simulink model "DeVriesSlipModelRW"  (R2017b)
settings: Solver=VariableStepAuto  StartTime=0.0  StopTime=100  RelTol=1e-3
undefined symbols (not defined in the file): b_contact, C_F_alpha, C_F_kappa, Cylinder, epsilon, g, k_contact, lengthRW, mR, Parts_Lib, radiusRW, rhoRW, sigma, X, xPla, Y, yPla, Z
libraries: nesl_utility x16, sm_lib x11, Contact_Forces_Lib x8, vrlib x2, dspsrcs4 x1, simulink x1
settings Model: Creator=r_ahmed_afzal  LastModifiedBy=r_ahmed_afzal
settings SolverCC: ZeroCrossAlgorithm=Adaptive

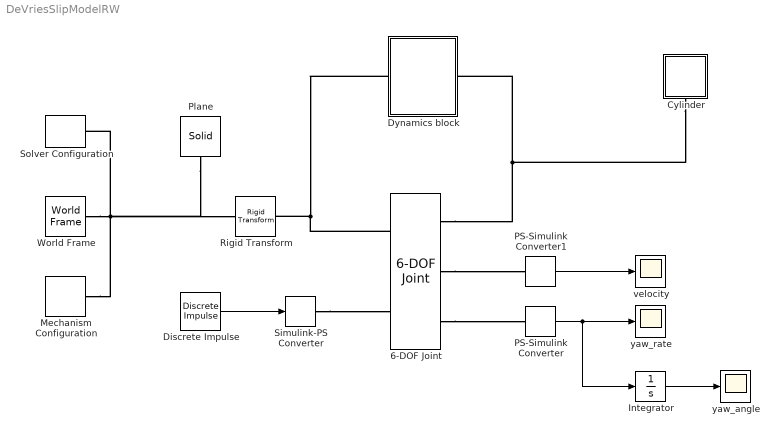
== system DeVriesSlipModelRW ==
  6-DOF Joint : sm_lib/Joints/6-DOF Joint  SenseConstraintForce=off  SenseConstraintForceX=off  SenseConstraintForceY=off  SenseConstraintForceZ=off  SenseConstraintTorque=off  SenseConstraintTorqueX=off  SenseConstraintTorqueY=off  SenseConstraintTorqueZ=off  SenseTotalForce=off  SenseTotalForceX=off  SenseTotalForceY=off  SenseTotalForceZ=off  SenseTotalTorque=off  SenseTotalTorqueX=off  SenseTotalTorqueY=off  SenseTotalTorqueZ=off  CompositeWrenchDir=FollowerOnBase  CompositeWrenchFrame=BaseFrame  PxEquilibriumPosition=0  PxEquilibriumPositionUnits=m  PxSpringStiffness=0  PxSpringStiffnessUnits=N/m  PxDampingCoefficient=0  PxDampingCoefficientUnits=N/(m/s)  PxTorqueActuationMode=NoTorque  PxMotionActuationMode=ComputedMotion  PxSensePosition=off  PxSenseVelocity=off  PxSenseAcceleration=off  PxSenseTorqueForce=off  PxPositionTargetSpecify=on  PxPositionTargetPriority=High  PxPositionTargetValue=radiusRW  PxPositionTargetValueUnits=m  PxVelocityTargetSpecify=off  PxVelocityTargetPriority=High  PxVelocityTargetValue=0  PxVelocityTargetValueUnits=m/s  PyEquilibriumPosition=0  PyEquilibriumPositionUnits=m  PySpringStiffness=0  PySpringStiffnessUnits=N/m  PyDampingCoefficient=0  PyDampingCoefficientUnits=N/(m/s)  PyTorqueActuationMode=NoTorque  PyMotionActuationMode=ComputedMotion  PySensePosition=off  PySenseVelocity=on  PySenseAcceleration=off  PySenseTorqueForce=off  PyPositionTargetSpecify=on  PyPositionTargetPriority=High  PyPositionTargetValue=-xPla/2 + 0.1  PyPositionTargetValueUnits=m  PyVelocityTargetSpecify=on  PyVelocityTargetPriority=High  PyVelocityTargetValue=v0  PyVelocityTargetValueUnits=m/s  PzEquilibriumPosition=0  PzEquilibriumPositionUnits=m  PzSpringStiffness=0  PzSpringStiffnessUnits=N/m  PzDampingCoefficient=0  PzDampingCoefficientUnits=N/(m/s)  PzTorqueActuationMode=NoTorque  PzMotionActuationMode=ComputedMotion  PzSensePosition=off  PzSenseVelocity=off  PzSenseAcceleration=off  PzSenseTorqueForce=off  PzPositionTargetSpecify=off  PzPositionTargetPriority=High  PzPositionTargetValue=0  PzPositionTargetValueUnits=m  PzVelocityTargetSpecify=off  PzVelocityTargetPriority=High  PzVelocityTargetValue=0  PzVelocityTargetValueUnits=m/s  SphDefPosRotationMethod=None  SphDefPosRotationAngleUnits=deg  SphDefPosRotationStandardAxis=+Z  SphDefPosRotationAngle=0.0  SphDefPosRotationArbitraryAxis=[0 0 1]  SphDefPosFollAlignAxisA=+X  SphDefPosBaseAlignAxisA=+Y  SphDefPosFollAlignAxisB=+Y  SphDefPosBaseAlignAxisB=+Z  SphDefPosRotationSequenceAxes=FollowerAxes  SphDefPosRotationSequence=XYX  SphDefPosRotationSequenceAngles=[0 0 0]  SphDefPosRotationSequenceAnglesUnits=deg  SphDefPosRotationMatrix=[1 0 0; 0 1 0; 0 0 1]  SphEqPosRotationMethod=None  SphEqPosRotationAngleUnits=deg  SphEqPosRotationStandardAxis=+Z  SphEqPosRotationAngle=0.0  SphEqPosRotationArbitraryAxis=[0 0 1]  SphEqPosFollAlignAxisA=+X  SphEqPosBaseAlignAxisA=+Y  SphEqPosFollAlignAxisB=+Y  SphEqPosBaseAlignAxisB=+Z  SphEqPosRotationSequenceAxes=FollowerAxes  SphEqPosRotationSequence=XYX  SphEqPosRotationSequenceAngles=[0 0 0]  SphEqPosRotationSequenceAnglesUnits=deg  SphEqPosRotationMatrix=[1 0 0; 0 1 0; 0 0 1]  SphSpringStiffness=0  SphSpringStiffnessUnits=N*m/deg  SphDampingCoefficient=0  SphDampingCoefficientUnits=N*m/(deg/s)  SphActuateTorqueX=off  SphActuateTorqueY=off  SphActuateTorqueZ=on  SphActuateTorque=off  SphTorqueActuationMode=InputTorque  SphMotionActuationMode=ComputedMotion  SphActuationFrame=FollowerFrame  SphSensePosition=off  SphSenseVelocityX=on  SphSenseVelocityY=off  SphSenseVelocityZ=off  SphSenseVelocity=off  SphSenseAccelerationX=off  SphSenseAccelerationY=off  SphSenseAccelerationZ=off  SphSenseAcceleration=off  SphSenseTorqueX=off  SphSenseTorqueY=off  SphSenseTorqueZ=off  SphSenseTorqueForce=off  SphSensingFrame=BaseFrame  SphPositionTargetRotationMethod=None  SphPositionTargetRotationAngleUnits=deg  SphPositionTargetRotationStandardAxis=+Z  SphPositionTargetRotationAngle=0.0  SphPositionTargetRotationArbitraryAxis=[0 0 1]  SphPositionTargetFollAlignAxisA=+X  SphPositionTargetBaseAlignAxisA=+Y  SphPositionTargetFollAlignAxisB=+Y  SphPositionTargetBaseAlignAxisB=+Z  SphPositionTargetRotationSequenceAxes=FollowerAxes  SphPositionTargetRotationSequence=XYX  SphPositionTargetRotationSequenceAngles=[0 0 0]  SphPositionTargetRotationSequenceAnglesUnits=deg  SphPositionTargetRotationMatrix=[1 0 0; 0 1 0; 0 0 1]  SphPositionTargetSpecify=off  SphPositionTargetPriority=High  SphVelocityTargetValue=[0 0 0]  SphVelocityTargetValueUnits=deg/s  SphVelocityTargetSpecify=off  SphVelocityTargetPriority=High  SphVelocityTargetInFollowerFrame=on
  Cylinder : Subsystem  Tag=CustomStyle  AncestorBlock=Parts_Lib/Cylinder  mask(Solid Cylinder with Markings){cyl_radius=radiusRW, cyl_length=lengthRW, cyl_density=rhoRW, cyl_color=blue, cyl_opacity=1, cyl_color_custom=[0.7920    0.9900    0.9900], mark_radius=[0.75 0.5], mark_len_factor=1.01, mark_angle=60, mark_color=purple, mark_opacity=1}
      mask prompts: cyl_radius "Radius (m)"; cyl_length "Length (m)"; cyl_density "Density (kg/m^3)"; cyl_color "Color"; cyl_opacity "Opacity (0-1)"; cyl_color_custom "Custom Color (rgb)"; mark_radius "Outer, inner radius (% of cylinder radius)"; mark_len_factor "Length (factor of cylinder length)"; mark_angle "Sweep angle (deg)"; mark_color "Color"; mark_opacity "Opacity (0-1)"
      mask init:
      | curblk = gcb;
      | if strcmp(get_param(curblk,'cyl_color'),'red')
      |     set_param([curblk '/Cylinder'],'GraphicDiffuseColor','[0.8 0.0 0.2]');
      |     set_param(curblk,'BackGroundColor','[0.901961, 0.396078, 0.396078]');
      | elseif strcmp(get_param(gcb,'cyl_color'),'blue')
      |     set_param([curblk '/Cylinder'],'GraphicDiffuseColor','[0.0 0.5 0.7]');
      |     set_param(curblk,'BackGroundColor','[0.541176, 0.698039, 0.901961]');
      | elseif strcmp(get_param(gcb,'cyl_color'),'yellow')
      |     set_param([curblk '/Cylinder'],'GraphicDiffuseColor','[1.0 1.0 0.0]');
      |     set_param(curblk,'BackGroundColor','[0.905882, 0.890196, 0.392157]');
      | elseif strcmp(get_param(gcb,'cyl_color'),'gray')
      |     set_param([curblk '/Cylinder'],'GraphicDiffuseColor','[1.0 1.0 1.0]*0.6');
      |     set_param(curblk,'BackGroundColor','[0.6 0.6 0.6]');
      | elseif strcmp(get_param(gcb,'cyl_color'),'custom')
      |     set_param([curblk '/Cylinder'],'GraphicDiffuseColor',get_param(curblk,'cyl_color_custom'));
      |     set_param(curblk,'BackGroundColor','[1 1 1]');
      | end
      | 
      | if strcmp(get_param(curblk,'mark_color'),'purple')
      |     set_param([curblk '/Vis1'],'GraphicDiffuseColor','[0.4 0.0 0.4]');
      |     set_param([curblk '/Vis2'],'GraphicDiffuseColor','[0.4 0.0 0.4]');
      | elseif strcmp(get_param(gcb,'mark_color'),'green')
      |     set_param([curblk '/Vis1'],'GraphicDiffuseColor','[0.0 0.8 0.0]');
      |     set_param([curblk '/Vis2'],'GraphicDiffuseColor','[0.0 0.8 0.0]');
      | elseif strcmp(get_param(gcb,'mark_color'),'orange')
      |     set_param([curblk '/Vis1'],'GraphicDiffuseColor','[1.0 0.6 0.0]');
      |     set_param([curblk '/Vis2'],'GraphicDiffuseColor','[1.0 0.6 0.0]');
      | elseif strcmp(get_param(gcb,'mark_color'),'black')
      |     set_param([curblk '/Vis1'],'GraphicDiffuseColor','[0.0 0.0 0.0]');
      |     set_param([curblk '/Vis2'],'GraphicDiffuseColor','[0.0 0.0 0.0]');
      | end
      | 
      | clear curblk
      mask TypeOptions cyl_color: red | gray | yellow | blue | custom
      mask Callback cyl_color:
      | maskObj = Simulink.Mask.get(gcb);
      | clr_h = maskObj.getParameter('cyl_color_custom');
      | if strcmp(get_param(gcb,'cyl_color'),'custom')
      |     clr_h.Visible = 'on';
      | else
      |     clr_h.Visible = 'off';
      | end
      mask TypeOptions mark_color: purple | green | orange | black
      mask DialogControl Container4 Prompt: Cylinder
      mask DialogControl Container7 Prompt: Markings
  Discrete Impulse : dspsrcs4/Discrete  Impulse  Delay=100  SampleTime=1  FrameSample=1  OutputFrames=off  dataType=double  isSigned=on  wordLen=16  udDataType=sfix(16)  fracBitsMode=Best precision  numFracBits=15  OutDataTypeStr=double  LastOutDataTypeStr=double
  Dynamics block : Subsystem
  Integrator : Integrator
  Mechanism Configuration : sm_lib/Utilities/Mechanism Configuration  UniformGravity=Constant  GravityVector=[0 0 -g]  GravityUnits=m/s^2  LinearizationDelta=0.001
  PS-Simulink Converter : nesl_utility/PS-Simulink Converter  PhysicalDomain=network_engine_domain  SubClassName=ps_output  LeftPortType=input  RightPortType=output  PseudoPeriodic=off  Frequencies=[]  Unit=1  AffineConversion=off
  PS-Simulink Converter1 : nesl_utility/PS-Simulink Converter  PhysicalDomain=network_engine_domain  SubClassName=ps_output  LeftPortType=input  RightPortType=output  PseudoPeriodic=off  Frequencies=[]  Unit=1  AffineConversion=off
  Plane : sm_lib/Body Elements/Solid  InertiaType=CalculateFromGeometry  Mass=1  MassUnits=kg  CenterOfMass=[0 0 0]  CenterOfMassUnits=m  MomentsOfInertia=[1 1 1]  MomentsOfInertiaUnits=kg*m^2  ProductsOfInertia=[1 1 1]  ProductsOfInertiaUnits=kg*m^2  DensityBased=on  Density=1000  DensityUnits=kg/m^3  DoExposeReferenceFrame=on  SerializedFrames=<Frames/>  GraphicType=FromGeometry  MarkerShape=Sphere  MarkerSize=10  GraphicVisPropType=SimpleVisualProperties  GraphicDiffuseColor=[0.5 0.5 0.5]  GraphicSpecularColor=[0.5 0.5 0.5 1.0]  GraphicAmbientColor=[0.15 0.15 0.15 1.0]  GraphicEmissiveColor=[0.0 0.0 0.0 1.0]  GraphicShininess=75  GraphicOpacity=0.5  GeometryShape=Brick  RectangleSize=[1 1]  RectangleSizeUnits=m  BrickDimensions=[xPla yPla 0.01]  BrickDimensionUnits=m  CylinderRadius=1  CylinderRadiusUnits=m  CylinderLength=1  CylinderLengthUnits=m  SphereRadius=1  SphereRadiusUnits=m  EllipsoidRadii=[1 1 1]  EllipsoidRadiiUnits=m  ExtrusionCrossSection=[1 1; -1 1; -1 -1; 1 -1]  ExtrusionCrossSectionUnits=m  ExtrusionLength=1  ExtrusionLengthUnits=m  PolygonNumSides=3  PolygonOuterRadius=1  PolygonOuterRadiusUnits=m  ExtGeomFileType=STEP  ExtGeomFileUnits=m  RevolutionCrossSection=[1 1; 1 -1; 2 -1; 2 1]  RevolutionCrossSectionUnits=m  RevolutionExtent=Full  RevolutionAngle=180  RevolutionAngleUnits=deg
  Rigid Transform : sm_lib/Frames and Transforms/Rigid Transform  TranslationMethod=None  TranslationStandardOffset=0  TranslationLengthUnit=m  TranslationStandardAxis=+Z  TranslationCartesianOffset=[0 0 0]  TranslationROffset=0  TranslationROffsetUnits=m  TranslationZOffset=0  TranslationZOffsetUnits=m  TranslationThetaOffset=0  TranslationThetaOffsetUnits=deg  RotationMethod=AlignedAxes  RotationAngleUnits=deg  RotationStandardAxis=+Z  RotationAngle=0.0  RotationArbitraryAxis=[0 0 1]  FollAlignAxisA=+Z  BaseAlignAxisA=+Y  FollAlignAxisB=+Y  BaseAlignAxisB=+X  RotationSequenceAxes=FollowerAxes  RotationSequence=XYX  RotationSequenceAngles=[0 0 0]  RotationSequenceAnglesUnits=deg  RotationMatrix=[1 0 0; 0 1 0; 0 0 1]
  Simulink-PS Converter : nesl_utility/Simulink-PS Converter  PhysicalDomain=network_engine_domain  SubClassName=ps_input  LeftPortType=input  RightPortType=output  PseudoPeriodic=off  Frequencies=[]  NoiseDistribution=none  NoiseParameters=[]  Unit=1  AffineConversion=off  FilteringAndDerivatives=provide  SimscapeFilterOrder=1  InputFilterTimeConstant=0.001  UdotUserProvided=0
  Solver Configuration : nesl_utility/Solver Configuration  PhysicalDomain=network_engine_domain  SubClassName=solver  LeftPortType=input  RightPortType=generic  Accelerate=off  Tones=[]  Harmonics=[]  SimulateNoise=off  Profile=off  UseLocalSampling=off  EnableSwitchedLinearOptims=on  FrequencyDomain=off  UseCCode=off  RelTol=0.001  AbsTol=1e-06  MinStep=1e-09  ToWorkspace=off  RevertToSquareIcSolve=off  NumHomotopyIterations=100  PhasorMode=off  PhasorModeNumHarmonics=1  DoDC=off  ResidualTolerance=1e-09  UseLocalSolver=off  LocalSolverChoice=NE_BACKWARD_EULER_ADVANCER  LocalSolverSampleTime=0.001  DoFixedCost=off  MaxNonlinIter=3  MaxModeIter=2  LinearAlgebra=Sparse  DelaysMemoryBudget=1024  AutomaticFiltering=on  FilteringTimeConstant=0.001
  World Frame : sm_lib/Frames and Transforms/World Frame
  velocity : Scope
  yaw_angle : Scope
  yaw_rate : Scope
  wires:
  Integrator/1 -> yaw_angle/1
  PS-Simulink Converter1/1 -> velocity/1
  PS-Simulink Converter/1 -> Integrator/1, yaw_rate/1
  Discrete Impulse/1 -> Simulink-PS Converter/1
  connections:
  Mechanism Configuration/RConn1 -- World Frame/RConn1 -- Rigid Transform/LConn1 -- Plane/RConn1 -- Solver Configuration/RConn1
  Dynamics block/LConn1 -- 6-DOF Joint/LConn1 -- Rigid Transform/RConn1
  Cylinder/LConn1 -- 6-DOF Joint/RConn1 -- Dynamics block/RConn1
  6-DOF Joint/RConn2 -- PS-Simulink Converter1/LConn1
  6-DOF Joint/RConn3 -- PS-Simulink Converter/LConn1
  Simulink-PS Converter/RConn1 -- 6-DOF Joint/LConn2

== system DeVriesSlipModelRW/Cylinder ==
  Cylinder : sm_lib/Body Elements/Solid  InertiaType=CalculateFromGeometry  Mass=mR  MassUnits=kg  CenterOfMass=[0 0 0]  CenterOfMassUnits=m  MomentsOfInertia=momentInertiaRW  MomentsOfInertiaUnits=kg*m^2  ProductsOfInertia=[0 0 0]  ProductsOfInertiaUnits=kg*m^2  DensityBased=on  Density=cyl_density  DensityUnits=kg/(m^3)  DoExposeReferenceFrame=on  SerializedFrames=<Frames/>  GraphicType=FromGeometry  MarkerShape=Sphere  MarkerSize=10  MarkerSizeUnits=m  GraphicVisPropType=SimpleVisualProperties  GraphicDiffuseColor=[0.0 0.5 0.7]  GraphicSpecularColor=[0.5 0.5 0.5 1.0]  GraphicAmbientColor=[0.15 0.15 0.15 1.0]  GraphicEmissiveColor=[0.0 0.0 0.0 1.0]  GraphicShininess=75  GraphicOpacity=cyl_opacity  GeometryShape=Cylinder  RectangleSize=[1 1]  RectangleSizeUnits=m  BrickDimensions=[1 1 1]  BrickDimensionUnits=m  CylinderRadius=cyl_radius  CylinderRadiusUnits=m  CylinderLength=cyl_length  CylinderLengthUnits=m  SphereRadius=1  SphereRadiusUnits=m  EllipsoidRadii=[1 1 1]  EllipsoidRadiiUnits=m  ExtrusionCrossSection=[1 1; -1 1; -1 -1; 1 -1]  ExtrusionCrossSectionUnits=m  ExtrusionLength=1  ExtrusionLengthUnits=m  PolygonNumSides=3  PolygonOuterRadius=1  PolygonOuterRadiusUnits=m  ExtGeomFileType=STL  ExtGeomFileUnits=m  RevolutionCrossSection=[1 1; 1 -1; 2 -1; 2 1]  RevolutionCrossSectionUnits=m  RevolutionExtent=Full  RevolutionAngle=180  RevolutionAngleUnits=deg
  Transform Vis2 : sm_lib/Frames and Transforms/Rigid Transform  TranslationMethod=None  TranslationStandardOffset=0  TranslationLengthUnit=m  TranslationStandardAxis=+Z  TranslationCartesianOffset=[0 0 0]  TranslationROffset=0  TranslationROffsetUnits=m  TranslationZOffset=0  TranslationZOffsetUnits=m  TranslationThetaOffset=0  TranslationThetaOffsetUnits=deg  RotationMethod=StandardAxis  RotationAngleUnits=deg  RotationStandardAxis=+Y  RotationAngle=180  RotationArbitraryAxis=[0 0 1]  FollAlignAxisA=+X  BaseAlignAxisA=+Y  FollAlignAxisB=+Y  BaseAlignAxisB=+Z  RotationSequenceAxes=FollowerAxes  RotationSequence=XYX  RotationSequenceAngles=[0 0 0]  RotationSequenceAnglesUnits=deg  RotationMatrix=[1 0 0; 0 1 0; 0 0 1]
  Vis1 : sm_lib/Body Elements/Solid  InertiaType=CalculateFromGeometry  Mass=1  MassUnits=kg  CenterOfMass=[0 0 0]  CenterOfMassUnits=m  MomentsOfInertia=[1 1 1]  MomentsOfInertiaUnits=kg*m^2  ProductsOfInertia=[0 0 0]  ProductsOfInertiaUnits=kg*m^2  DensityBased=on  Density=1e-3  DensityUnits=kg/(m^3)  DoExposeReferenceFrame=on  SerializedFrames=<Frames/>  GraphicType=FromGeometry  MarkerShape=Sphere  MarkerSize=10  MarkerSizeUnits=m  GraphicVisPropType=SimpleVisualProperties  GraphicDiffuseColor=[0.4 0.0 0.4]  GraphicSpecularColor=[0.5 0.5 0.5 1.0]  GraphicAmbientColor=[0.15 0.15 0.15 1.0]  GraphicEmissiveColor=[0.0 0.0 0.0 1.0]  GraphicShininess=75  GraphicOpacity=mark_opacity  GeometryShape=GeneralSolidOfRevolution  RectangleSize=[1 1]  RectangleSizeUnits=m  BrickDimensions=[1 1 1]  BrickDimensionUnits=m  CylinderRadius=0.1  CylinderRadiusUnits=m  CylinderLength=0.01  CylinderLengthUnits=m  SphereRadius=1  SphereRadiusUnits=m  EllipsoidRadii=[1 1 1]  EllipsoidRadiiUnits=m  ExtrusionCrossSection=[1 1; -1 1; -1 -1; 1 -1]  ExtrusionCrossSectionUnits=m  ExtrusionLength=1  ExtrusionLengthUnits=m  PolygonNumSides=3  PolygonOuterRadius=1  PolygonOuterRadiusUnits=m  ExtGeomFileType=STL  ExtGeomFileUnits=m  RevolutionCrossSection=[cyl_radius*mark_radius(1) cyl_length/2*mark_len_factor; cyl_radius*mark_radius(2) cyl_length/2*mark_len_factor; cyl_radius*mark_radius(2) -cyl_length/2*mark_len_factor; cyl_radius*mark_radius(1) -cyl_length/2*mark_len_factor]  RevolutionCrossSectionUnits=m  RevolutionExtent=Custom  RevolutionAngle=mark_angle  RevolutionAngleUnits=deg
  Vis2 : sm_lib/Body Elements/Solid  InertiaType=CalculateFromGeometry  Mass=1  MassUnits=kg  CenterOfMass=[0 0 0]  CenterOfMassUnits=m  MomentsOfInertia=[1 1 1]  MomentsOfInertiaUnits=kg*m^2  ProductsOfInertia=[0 0 0]  ProductsOfInertiaUnits=kg*m^2  DensityBased=on  Density=1e-3  DensityUnits=kg/(m^3)  DoExposeReferenceFrame=on  SerializedFrames=<Frames/>  GraphicType=FromGeometry  MarkerShape=Sphere  MarkerSize=10  MarkerSizeUnits=m  GraphicVisPropType=SimpleVisualProperties  GraphicDiffuseColor=[0.4 0.0 0.4]  GraphicSpecularColor=[0.5 0.5 0.5 1.0]  GraphicAmbientColor=[0.15 0.15 0.15 1.0]  GraphicEmissiveColor=[0.0 0.0 0.0 1.0]  GraphicShininess=75  GraphicOpacity=mark_opacity  GeometryShape=GeneralSolidOfRevolution  RectangleSize=[1 1]  RectangleSizeUnits=m  BrickDimensions=[1 1 1]  BrickDimensionUnits=m  CylinderRadius=0.1  CylinderRadiusUnits=m  CylinderLength=0.01  CylinderLengthUnits=m  SphereRadius=1  SphereRadiusUnits=m  EllipsoidRadii=[1 1 1]  EllipsoidRadiiUnits=m  ExtrusionCrossSection=[1 1; -1 1; -1 -1; 1 -1]  ExtrusionCrossSectionUnits=m  ExtrusionLength=1  ExtrusionLengthUnits=m  PolygonNumSides=3  PolygonOuterRadius=1  PolygonOuterRadiusUnits=m  ExtGeomFileType=STL  ExtGeomFileUnits=m  RevolutionCrossSection=[cyl_radius*mark_radius(1) cyl_length/2*mark_len_factor; cyl_radius*mark_radius(2) cyl_length/2*mark_len_factor; cyl_radius*mark_radius(2) -cyl_length/2*mark_len_factor; cyl_radius*mark_radius(1) -cyl_length/2*mark_len_factor]  RevolutionCrossSectionUnits=m  RevolutionExtent=Custom  RevolutionAngle=mark_angle  RevolutionAngleUnits=deg
  R : PMIOPort  Port=1  Side=Left
  connections:
  R/RConn1 -- Cylinder/RConn1 -- Transform Vis2/LConn1 -- Vis1/RConn1
  Vis2/RConn1 -- Transform Vis2/RConn1

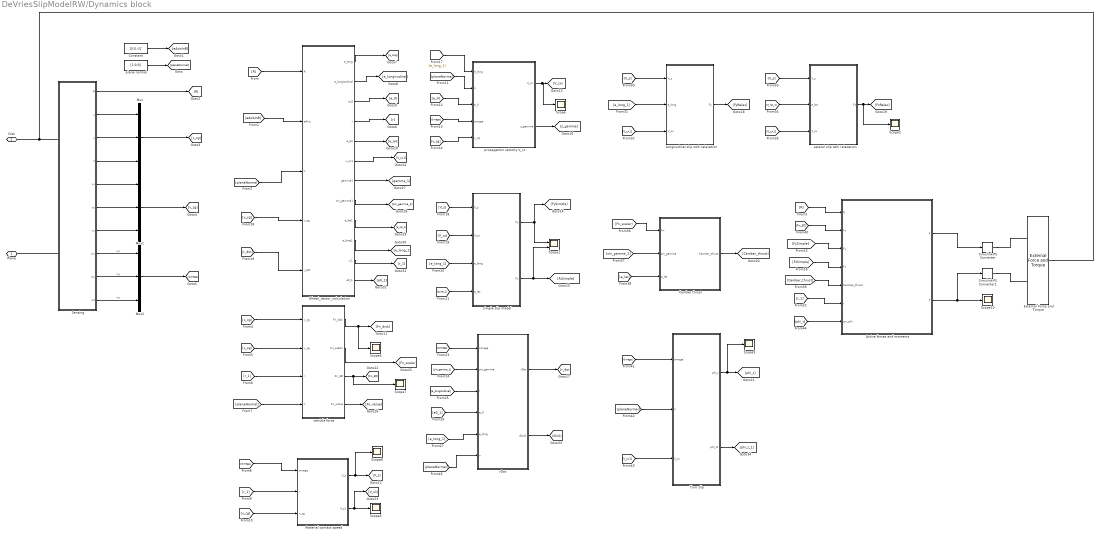
== system DeVriesSlipModelRW/Dynamics block ==
  Active forces and moments : Subsystem
  Camber thrust : Subsystem
  Constant : Constant  Value=[0,0,-1]'
  External Force and Torque : sm_lib/Forces and Torques/External Force and Torque  ForceResolutionFrame=AttachedFrame  EnableForceX=off  EnableForceY=off  EnableForceZ=off  EnableForce=on  TorqueResolutionFrame=AttachedFrame  EnableTorqueX=off  EnableTorqueY=off  EnableTorqueZ=off  EnableTorque=on
  Lateral slip wtih relaxation : Subsystem
  Longitudinal slip wtih relaxation : Subsystem
  Material contact speed : Subsystem
  Mux : Mux  Inputs=3
  Mux1 : Mux  Inputs=3
  Mux2 : Mux  Inputs=3
  Scope{,2,4..7,9..10} (8 alike) : Scope
  Scope1 : Scope  NumInputPorts=2
  Sensing : Subsystem
  Simulink-PS Converter : nesl_utility/Simulink-PS Converter  PhysicalDomain=network_engine_domain  SubClassName=ps_input  LeftPortType=input  RightPortType=output  PseudoPeriodic=off  Frequencies=[]  NoiseDistribution=none  NoiseParameters=[]  Unit=1  AffineConversion=off  FilteringAndDerivatives=provide  SimscapeFilterOrder=1  InputFilterTimeConstant=0.001  UdotUserProvided=0
  Simulink-PS Converter1 : nesl_utility/Simulink-PS Converter  PhysicalDomain=network_engine_domain  SubClassName=ps_input  LeftPortType=input  RightPortType=output  PseudoPeriodic=off  Frequencies=[]  NoiseDistribution=none  NoiseParameters=[]  Unit=1  AffineConversion=off  FilteringAndDerivatives=provide  SimscapeFilterOrder=1  InputFilterTimeConstant=0.001  UdotUserProvided=0
  Turn slip : Subsystem
  Wheel_vector_calculation : Subsystem
  plane normal : Constant  Value=[1;0;0]
  propagation velocity V_cx : Subsystem
  rDot : Subsystem
  simple slip model : Subsystem
  verticle force : Subsystem
  Plane : PMIOPort  Port=1  Side=Left
  Disk : PMIOPort  Port=2  Side=Right
  wires:
  plane normal/1 -> [planeNormal]
  Constant/1 -> [eAxisInB]
  Sensing/1(R) -> [R]
  Sensing/2(x) -> Mux/1
  Sensing/3(y) -> Mux/2
  Sensing/4(z) -> Mux/3
  Mux/1 -> [x_cg]
  Sensing/6(vy) -> Mux1/2
  Sensing/5(vx) -> Mux1/1
  Sensing/7(vz) -> Mux1/3
  Mux1/1 -> [v_cg]
  Sensing/9(wy) -> Mux2/2  "wy"
  Sensing/8(wx) -> Mux2/1  "wx"
  Sensing/10(wz) -> Mux2/3  "wz"
  [R] -> Wheel_vector_calculation/1(R)
  [planeNormal] -> Wheel_vector_calculation/3(n)
  [x_cg] -> verticle force/1(x_cg)
  [v_cg] -> verticle force/2(v_cg)
  Wheel_vector_calculation/4(r) -> [r]
  Wheel_vector_calculation/1(e_long) -> [e_long]
  Wheel_vector_calculation/2(e_longitudinal) -> [e_longitudinal]
  Wheel_vector_calculation/3(e_0) -> [e_0]
  Wheel_vector_calculation/5(e_lat) -> [e_lat]
  [r_1] -> verticle force/3(r)
  [planeNormal] -> verticle force/4(n)
  verticle force/1(Fn_disk) -> Scope4/1, [Fn_disk]
  [Omega] -> Material contact speed/1(omega)
  [r_1] -> Material contact speed/2(r)
  [v_cg] -> Material contact speed/3(v_cg)
  Material contact speed/1(V_s) -> Scope6/1, [V_s]
  [planeNormal] -> propagation velocity V_cx/2(n)
  [e_0] -> propagation velocity V_cx/3(e_0)
  [Omega] -> propagation velocity V_cx/4(omega)
  [v_cg] -> propagation velocity V_cx/5(v_cg)
  [e_long_1] -> propagation velocity V_cx/1(e_long)
  propagation velocity V_cx/1(V_cx) -> Scope/1, [V_cx]
  [V_s] -> simple slip model/1(V_s)
  [V_cx] -> simple slip model/2(V_cx)
  [e_long_1] -> simple slip model/3(e_long)
  [e_lat_1] -> simple slip model/4(e_lat)
  simple slip model/2(Fz) -> Scope1/2, [FzSimple]
  [Omega] -> rDot/1(omega)
  propagation velocity V_cx/2(s_gamma) -> [s_gamma]
  [sin_gamma_1] -> rDot/2(sin_gamma)
  [e_longitudinal] -> rDot/3(l)
  [e0_1] -> rDot/4(e_0)
  [e_long_1] -> rDot/5(e_long)
  simple slip model/1(Fy) -> [FySimple], Scope1/1
  [V_s] -> Longitudinal slip wtih relaxation/1(V_s)
  [e_long_1] -> Longitudinal slip wtih relaxation/2(e_long)
  [V_cx1] -> Longitudinal slip wtih relaxation/3(V_cx)
  [e_lat_1] -> Lateral slip wtih relaxation/2(e_lat)
  [V_s] -> Lateral slip wtih relaxation/1(V_s)
  [V_cx1] -> Lateral slip wtih relaxation/3(V_cx)
  Longitudinal slip wtih relaxation/1(Fy) -> [FyRelax]
  Lateral slip wtih relaxation/1(Fz) -> Scope2/1, [FzRelax]
  [Fn_scalar] -> Camber thrust/1(Fn)
  [sin_gamma_1] -> Camber thrust/2(sin_gamma)
  [e_lat] -> Camber thrust/3(e_lat)
  Camber thrust/1(Camber_thrust) -> [Camber_thrust]
  Turn slip/1(phi_t) -> Scope9/1, [phi_t]
  [V_cx1] -> Turn slip/3(V_cx)
  [planeNormal] -> Turn slip/2(n)
  [Omega] -> Turn slip/1(omega)
  [R] -> Active forces and moments/1(R)
  [Fn_3D] -> Active forces and moments/2(Fx)
  [FySimple] -> Active forces and moments/3(Fy)
  [r_1] -> Active forces and moments/6(r)
  Active forces and moments/1(F) -> Simulink-PS Converter/1
  Active forces and moments/2(T) -> Scope10/1, Simulink-PS Converter1/1
  verticle force/3(Fn_3D) -> [Fn_3D], Scope7/1
  verticle force/2(Fn_scalar) -> [Fn_scalar]
  [v_cg] -> Wheel_vector_calculation/4(v_cg)
  rDot/1(rDot) -> [r_dot]
  [r_dot] -> Wheel_vector_calculation/5(r_dot)
  Wheel_vector_calculation/6(v_cx1) -> [V_cx1]
  Mux2/1 -> [Omega]
  Material contact speed/2(V_s1) -> [V_s1], Scope5/1
  verticle force/4(Fn_value) -> [Fn_value]
  [eAxisInB] -> Wheel_vector_calculation/2(eAxis)
  [Camber_thrust] -> Active forces and moments/5(Camber_thrust)
  [phi_t] -> Active forces and moments/7(cm_phi)
  Wheel_vector_calculation/7(gamma1) -> [gamma_1]
  Wheel_vector_calculation/8(sin_gamma1) -> [sin_gamma_1]
  Wheel_vector_calculation/9(e_lat1) -> [e_lat_1]
  Wheel_vector_calculation/10(e_long1) -> [e_long_1]
  Wheel_vector_calculation/11(r_1) -> [r_1]
  Wheel_vector_calculation/12(e0_1) -> [e0_1]
  [planeNormal] -> rDot/6(n)
  rDot/2(rDot1) -> [rDot1]
  Turn slip/2(phi_t1) -> [phi_t_1]
  [FzSimple] -> Active forces and moments/4(Fz)
  connections:
  Sensing/LConn1 -- External Force and Torque/RConn1 -- Disk/RConn1
  Sensing/LConn2 -- Plane/RConn1
  Simulink-PS Converter/RConn1 -- External Force and Torque/LConn1
  Simulink-PS Converter1/RConn1 -- External Force and Torque/LConn2

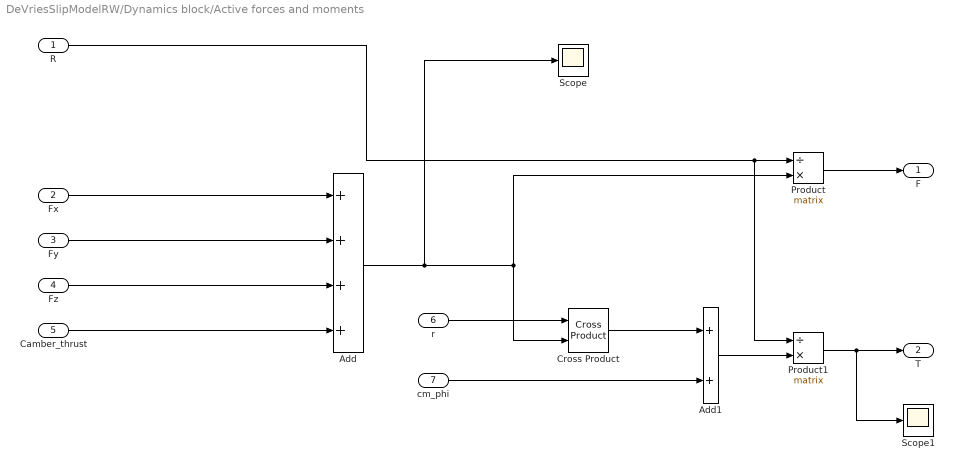
== system DeVriesSlipModelRW/Dynamics block/Active forces and moments ==
  R : Inport
  Fx : Inport  Port=2
  Fy : Inport  Port=3
  Fz : Inport  Port=4
  Camber_thrust : Inport  Port=5
  r : Inport  Port=6
  cm_phi : Inport  Port=7
  Add : Sum  Inputs=4
  Add1 : Sum
  Cross Product : Contact_Forces_Lib/Math/Cross Product
  Product : Product  Inputs=/*  Multiplication=Matrix(*)
  Product1 : Product  Inputs=/*  Multiplication=Matrix(*)
  Scope : Scope
  Scope1 : Scope
  F : Outport
  T : Outport  Port=2
  wires:
  Fy/1 -> Add/2
  R/1 -> Product1/1, Product/1
  Fx/1 -> Add/1
  Camber_thrust/1 -> Add/4
  Add/1 -> Scope/1, Cross Product/2, Product/2
  Product/1 -> F/1
  cm_phi/1 -> Add1/2
  Cross Product/1 -> Add1/1
  Add1/1 -> Product1/2
  Product1/1 -> Scope1/1, T/1
  r/1 -> Cross Product/1
  Fz/1 -> Add/3

== system DeVriesSlipModelRW/Dynamics block/Camber thrust ==
  Fn : Inport
  sin_gamma : Inport  Port=2
  e_lat : Inport  Port=3
  Product : Product
  Product1 : Product
  Scope : Scope
  Camber_thrust : Outport
  wires:
  Fn/1 -> Product/1
  sin_gamma/1 -> Product/2
  Product/1 -> Scope/1, Product1/1
  e_lat/1 -> Product1/2
  Product1/1 -> Camber_thrust/1

== system DeVriesSlipModelRW/Dynamics block/Lateral slip wtih relaxation ==
  V_s : Inport
  e_lat : Inport  Port=2
  V_cx : Inport  Port=3
  Dot Product : DotProduct  InputSameDT=on  OutDataTypeStr=Inherit: Inherit via internal rule
  Gain : Gain  Gain=1/sigma
  Gain1 : Gain  Gain=-C_F_alpha
  Integrator : Integrator
  Product : Product
  Product1 : Product
  Scope : Scope
  Sum : Sum  Inputs=|+-
  Fz : Outport
  wires:
  V_s/1 -> Dot Product/1
  e_lat/1 -> Product1/2, Dot Product/2
  Dot Product/1 -> Sum/1
  Sum/1 -> Gain/1
  Gain/1 -> Integrator/1
  Integrator/1 -> Scope/1, Product/2, Gain1/1
  Gain1/1 -> Product1/1
  Product/1 -> Sum/2
  V_cx/1 -> Product/1
  Product1/1 -> Fz/1

== system DeVriesSlipModelRW/Dynamics block/Longitudinal slip wtih relaxation ==
  V_s : Inport
  e_long : Inport  Port=2
  V_cx : Inport  Port=3
  Dot Product : DotProduct  InputSameDT=on  OutDataTypeStr=Inherit: Inherit via internal rule
  Gain : Gain  Gain=1/sigma
  Gain1 : Gain  Gain=-C_F_kappa
  Integrator : Integrator
  Product : Product
  Product1 : Product
  Scope : Scope
  Sum : Sum  Inputs=|+-
  Fy : Outport
  wires:
  V_s/1 -> Dot Product/1
  e_long/1 -> Product1/2, Dot Product/2
  Dot Product/1 -> Sum/1
  Sum/1 -> Gain/1
  Gain/1 -> Integrator/1
  Integrator/1 -> Product/2, Gain1/1
  Gain1/1 -> Product1/1
  Product/1 -> Sum/2
  V_cx/1 -> Product/1
  Product1/1 -> Scope/1, Fy/1

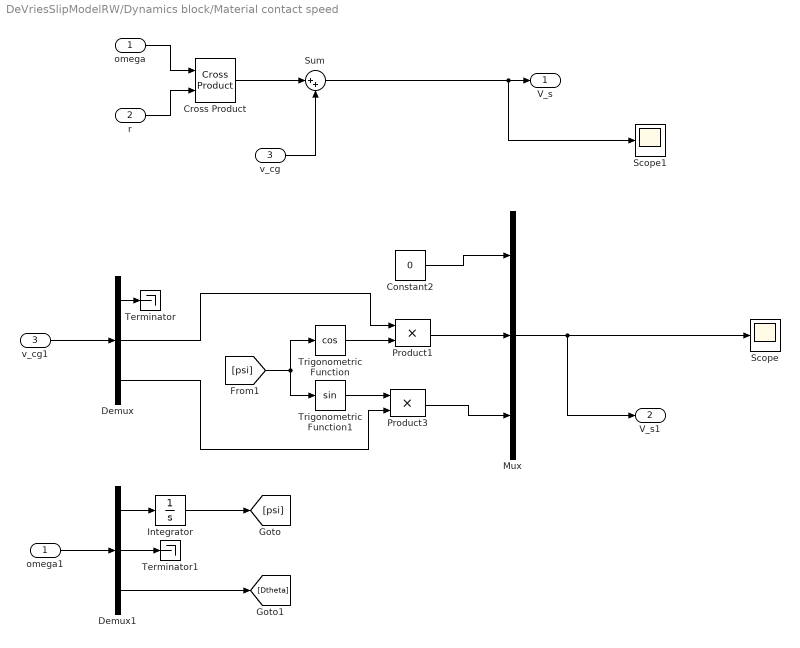
== system DeVriesSlipModelRW/Dynamics block/Material contact speed ==
  omega : Inport
  r : Inport  Port=2
  v_cg : Inport  Port=3
  Constant2 : Constant  Value=0
  Cross Product : Contact_Forces_Lib/Math/Cross Product
  Demux : Demux  Outputs=3
  Demux1 : Demux  Outputs=3
  Integrator : Integrator
  Mux : Mux  Inputs=3
  Product1 : Product  SaturateOnIntegerOverflow=on  InputSameDT=on  OutDataTypeStr=Inherit: Same as first input
  Product3 : Product  SaturateOnIntegerOverflow=on  InputSameDT=on  OutDataTypeStr=Inherit: Same as first input
  Scope : Scope
  Scope1 : Scope
  Sum : Sum  Inputs=|++
  Terminator : Terminator
  Terminator1 : Terminator
  Trigonometric Function : Trigonometry  Operator=cos
  Trigonometric Function1 : Trigonometry
  omega1 : InportShadow
  v_cg1 : InportShadow  Port=3
  V_s : Outport
  V_s1 : Outport  Port=2
  wires:
  omega/1 -> Cross Product/1
  r/1 -> Cross Product/2
  Cross Product/1 -> Sum/1
  v_cg/1 -> Sum/2
  Sum/1 -> Scope1/1, V_s/1
  Trigonometric Function/1 -> Product1/2
  Demux/2 -> Product1/1
  Trigonometric Function1/1 -> Product3/1
  Demux/3 -> Product3/2
  v_cg1/1 -> Demux/1
  Demux/1 -> Terminator/1
  omega1/1 -> Demux1/1
  Demux1/1 -> Integrator/1
  Demux1/2 -> Terminator1/1
  Demux1/3 -> [Dtheta]
  Integrator/1 -> [psi]
  [psi] -> Trigonometric Function/1, Trigonometric Function1/1
  Product1/1 -> Mux/2
  Product3/1 -> Mux/3
  Constant2/1 -> Mux/1
  Mux/1 -> V_s1/1, Scope/1

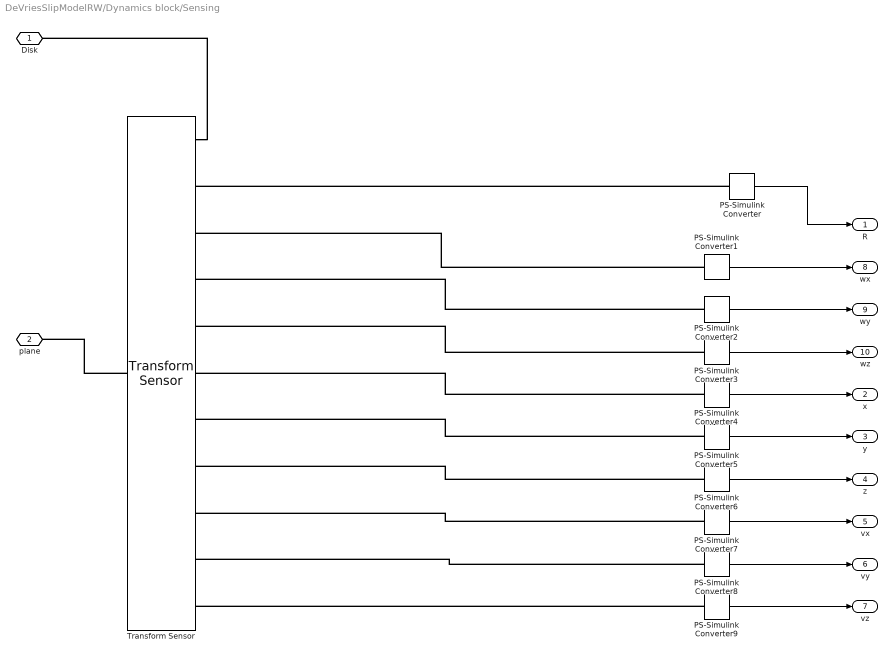
== system DeVriesSlipModelRW/Dynamics block/Sensing ==
  PS-Simulink Converter{,1..9} (10 alike) : nesl_utility/PS-Simulink Converter  PhysicalDomain=network_engine_domain  SubClassName=ps_output  LeftPortType=input  RightPortType=output  PseudoPeriodic=off  Frequencies=[]  Unit=1  AffineConversion=off
  Transform Sensor : sm_lib/Frames and Transforms/Transform Sensor  MeasurementFrame=Base  SenseAngle=off  SenseAxis=off  SenseAngle1=off  SenseAngle2=off  SenseAngle3=off  SenseQ=off  SenseR=on  SenseOmegaX=on  SenseOmegaY=on  SenseOmegaZ=on  SenseOmega1=off  SenseOmega2=off  SenseOmega3=off  SenseQDot=off  SenseRDot=off  SenseAlphaX=off  SenseAlphaY=off  SenseAlphaZ=off  SenseAlpha1=off  SenseAlpha2=off  SenseAlpha3=off  SenseQDDot=off  SenseRDDot=off  SenseX=on  SenseY=on  SenseZ=on  SenseRad=off  SenseAzim=off  SenseDist=off  SenseInc=off  SenseXDot=on  SenseYDot=on  SenseZDot=on  SenseRadDot=off  SenseAzimDot=off  SenseDistDot=off  SenseIncDot=off  SenseXDDot=off  SenseYDDot=off  SenseZDDot=off  SenseRadDDot=off  SenseAzimDDot=off  SenseDistDDot=off  SenseIncDDot=off
  Disk : PMIOPort  Port=1  Side=Left
  plane : PMIOPort  Port=2  Side=Left
  R : Outport
  x : Outport  Port=2
  y : Outport  Port=3
  z : Outport  Port=4
  vx : Outport  Port=5
  vy : Outport  Port=6
  vz : Outport  Port=7
  wx : Outport  Port=8
  wy : Outport  Port=9
  wz : Outport  Port=10
  wires:
  PS-Simulink Converter/1 -> R/1
  PS-Simulink Converter4/1 -> x/1
  PS-Simulink Converter7/1 -> vx/1
  PS-Simulink Converter9/1 -> vz/1
  PS-Simulink Converter5/1 -> y/1
  PS-Simulink Converter6/1 -> z/1
  PS-Simulink Converter1/1 -> wx/1
  PS-Simulink Converter3/1 -> wz/1
  PS-Simulink Converter8/1 -> vy/1
  PS-Simulink Converter2/1 -> wy/1
  connections:
  PS-Simulink Converter8/LConn1 -- Transform Sensor/RConn10
  PS-Simulink Converter9/LConn1 -- Transform Sensor/RConn11
  PS-Simulink Converter7/LConn1 -- Transform Sensor/RConn9
  PS-Simulink Converter2/LConn1 -- Transform Sensor/RConn4
  PS-Simulink Converter1/LConn1 -- Transform Sensor/RConn3
  PS-Simulink Converter6/LConn1 -- Transform Sensor/RConn8
  PS-Simulink Converter4/LConn1 -- Transform Sensor/RConn6
  PS-Simulink Converter5/LConn1 -- Transform Sensor/RConn7
  Transform Sensor/RConn1 -- Disk/RConn1
  Transform Sensor/LConn1 -- plane/RConn1
  PS-Simulink Converter/LConn1 -- Transform Sensor/RConn2
  PS-Simulink Converter3/LConn1 -- Transform Sensor/RConn5

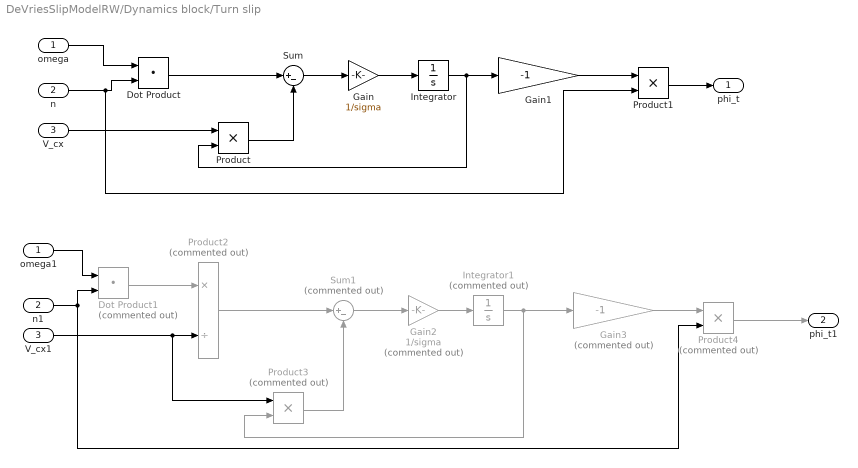
== system DeVriesSlipModelRW/Dynamics block/Turn slip ==
  omega : Inport
  n : Inport  Port=2
  V_cx : Inport  Port=3
  Dot Product : DotProduct  InputSameDT=on  OutDataTypeStr=Inherit: Inherit via internal rule
  Dot Product1 : DotProduct  Commented=on  InputSameDT=on  OutDataTypeStr=Inherit: Inherit via internal rule
  Gain : Gain  Gain=1/sigma
  Gain1 : Gain  Gain=-1
  Gain2 : Gain  Commented=on  Gain=1/sigma
  Gain3 : Gain  Commented=on  Gain=-1
  Integrator : Integrator
  Integrator1 : Integrator  Commented=on
  Product : Product
  Product1 : Product
  Product2 : Product  Commented=on  Inputs=*/
  Product3 : Product  Commented=on
  Product4 : Product  Commented=on
  Sum : Sum  Inputs=|+-
  Sum1 : Sum  Commented=on  Inputs=|+-
  V_cx1 : InportShadow  Port=3
  n1 : InportShadow  Port=2
  omega1 : InportShadow
  phi_t : Outport
  phi_t1 : Outport  Port=2
  wires:
  omega/1 -> Dot Product/1
  n/1 -> Product1/2, Dot Product/2
  Dot Product/1 -> Sum/1
  Sum/1 -> Gain/1
  Gain/1 -> Integrator/1
  Integrator/1 -> Product/2, Gain1/1
  Gain1/1 -> Product1/1
  Product1/1 -> phi_t/1
  Product/1 -> Sum/2
  V_cx/1 -> Product/1
  omega1/1 -> Dot Product1/1
  n1/1 -> Product4/2, Dot Product1/2
  Dot Product1/1 -> Product2/1
  V_cx1/1 -> Product3/1, Product2/2
  Product2/1 -> Sum1/1
  Sum1/1 -> Gain2/1
  Product3/1 -> Sum1/2
  Gain2/1 -> Integrator1/1
  Integrator1/1 -> Gain3/1, Product3/2
  Gain3/1 -> Product4/1
  Product4/1 -> phi_t1/1

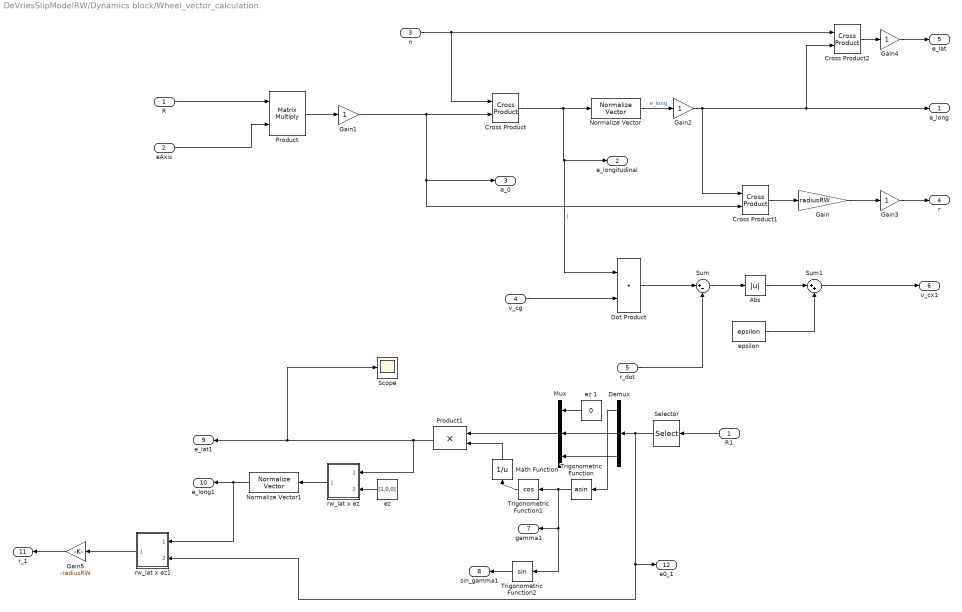
== system DeVriesSlipModelRW/Dynamics block/Wheel_vector_calculation ==
  R : Inport
  eAxis : Inport  Port=2
  n : Inport  Port=3
  v_cg : Inport  Port=4
  r_dot : Inport  Port=5
  Abs : Abs
  Cross Product : Contact_Forces_Lib/Math/Cross Product
  Cross Product1 : Contact_Forces_Lib/Math/Cross Product
  Cross Product2 : Contact_Forces_Lib/Math/Cross Product
  Demux : Demux  Outputs=3
  Dot Product : DotProduct  InputSameDT=on  OutDataTypeStr=Inherit: Inherit via internal rule
  Gain : Gain  Gain=radiusRW
  Gain{1..4} (4 alike) : Gain
  Gain5 : Gain  Gain=-radiusRW
  Math Function : Math  Operator=reciprocal  SaturateOnIntegerOverflow=on
  Mux : Mux  Inputs=3
  Normalize Vector : vrlib/Utilities/Normalize Vector  maxzero=0
      settings: SourceProductName=Simulink 3D Animation  SourceProductBaseCode=VR
  Normalize Vector1 : vrlib/Utilities/Normalize Vector  maxzero=0
      settings: SourceProductName=Simulink 3D Animation  SourceProductBaseCode=VR
  Product : Product  Multiplication=Matrix(*)
  Product1 : Product  SaturateOnIntegerOverflow=on  InputSameDT=on  OutDataTypeStr=Inherit: Same as first input
  R1 : InportShadow
  Scope : Scope
  Selector : Selector  NumberOfDimensions=2  InputPortWidth=9  IndexOptions=Select all,Index vector (dialog)  Indices=[4:6],3  OutputSizes=1,1
  Sum : Sum  Inputs=|+-
  Sum1 : Sum  Inputs=|++
  Trigonometric Function : Trigonometry  Operator=asin
  Trigonometric Function1 : Trigonometry  Operator=cos
  Trigonometric Function2 : Trigonometry
  epsilon : Constant  Value=epsilon
  "ez " : Constant  Value=[1,0,0]
  ez 1 : Constant  Value=0
  rw_lat x ez : Subsystem  mask(Cross Product){}
      mask help: Calculates the cross product of two 3x1 vectors.
      mask Help:
      | <p>This block calculates the cross product of two 3x1 vectors, ie.</p>
      | 
      | <ul>C(1) = A(2)*B(3) - A(3)*B(2)</ul>
      | <ul>C(2) = A(3)*B(1) - A(1)*B(3)</ul>
      | <ul>C(3) = A(1)*B(2) - A(2)*B(1)</ul>
      | 
      | <p>The block inputs and output contain more than one signal as described below.</p>
      | 
      | <p><H4>Block Vector Input 1 - A</H4>
      | <ul>
      | <li>A(1)</li>
      | <li>A(2)</li>
      | <li>A(3)</li>
      | </ul>
      | </p>
      | 
      | <p><H4>Block Vector Input 2 - B</H4>
      | <ul>
      | <li>B(1)</li>
      | <li>B(2)</li>
      | <li>B(3)</li>
      | </ul>
      | </p>
      | 
      | <p><H4>Block Vector Output - Cross Product (AxB)</H4>
      | <ul>
      | <li>C(1)</li>
      | <li>C(2)</li>
      | <li>C(3)</li>
      | </ul>
      | </p>
      mask Display: disp('Cross\nProduct')
  rw_lat x ez1 : Subsystem  mask(Cross Product){}
      mask help: Calculates the cross product of two 3x1 vectors.
      mask Help:
      | <p>This block calculates the cross product of two 3x1 vectors, ie.</p>
      | 
      | <ul>C(1) = A(2)*B(3) - A(3)*B(2)</ul>
      | <ul>C(2) = A(3)*B(1) - A(1)*B(3)</ul>
      | <ul>C(3) = A(1)*B(2) - A(2)*B(1)</ul>
      | 
      | <p>The block inputs and output contain more than one signal as described below.</p>
      | 
      | <p><H4>Block Vector Input 1 - A</H4>
      | <ul>
      | <li>A(1)</li>
      | <li>A(2)</li>
      | <li>A(3)</li>
      | </ul>
      | </p>
      | 
      | <p><H4>Block Vector Input 2 - B</H4>
      | <ul>
      | <li>B(1)</li>
      | <li>B(2)</li>
      | <li>B(3)</li>
      | </ul>
      | </p>
      | 
      | <p><H4>Block Vector Output - Cross Product (AxB)</H4>
      | <ul>
      | <li>C(1)</li>
      | <li>C(2)</li>
      | <li>C(3)</li>
      | </ul>
      | </p>
      mask Display: disp('Cross\nProduct')
  e_long : Outport
  e_longitudinal : Outport  Port=2
  e_0 : Outport  Port=3
  r : Outport  Port=4
  e_lat : Outport  Port=5
  v_cx1 : Outport  Port=6
  gamma1 : Outport  Port=7
  sin_gamma1 : Outport  Port=8
  e_lat1 : Outport  Port=9
  e_long1 : Outport  Port=10
  r_1 : Outport  Port=11
  e0_1 : Outport  Port=12
  wires:
  n/1 -> Cross Product/1, Cross Product2/1
  Cross Product/1 -> Dot Product/1, e_longitudinal/1, Normalize Vector/1  "l"
  Cross Product1/1 -> Gain/1
  Gain/1 -> Gain3/1
  Cross Product2/1 -> Gain4/1
  Gain1/1 -> Cross Product1/2, e_0/1, Cross Product/2
  Normalize Vector/1 -> Gain2/1  "e_long"
  Gain2/1 -> Cross Product1/1, Cross Product2/2, e_long/1
  Gain3/1 -> r/1
  v_cg/1 -> Dot Product/2
  Dot Product/1 -> Sum/1
  r_dot/1 -> Sum/2
  Sum/1 -> Abs/1
  Abs/1 -> Sum1/1
  epsilon/1 -> Sum1/2
  Sum1/1 -> v_cx1/1
  eAxis/1 -> Product/2
  Product/1 -> Gain1/1
  Gain4/1 -> e_lat/1
  R/1 -> Product/1
  Trigonometric Function/1 -> Trigonometric Function1/1, Trigonometric Function2/1, gamma1/1
  "ez "/1 -> rw_lat x ez/2(b(1) b(2) b(3))
  R1/1 -> Selector/1
  Product1/1 -> Scope/1, e_lat1/1, rw_lat x ez/1(a(1) a(2) a(3))
  Math Function/1 -> Product1/2
  Trigonometric Function1/1 -> Math Function/1
  Mux/1 -> Product1/1
  rw_lat x ez/1(c(1) c(2) c(3)) -> Normalize Vector1/1
  Trigonometric Function2/1 -> sin_gamma1/1
  rw_lat x ez1/1(c(1) c(2) c(3)) -> Gain5/1
  Selector/1 -> e0_1/1, rw_lat x ez1/2(b(1) b(2) b(3)), Demux/1
  Demux/1 -> Trigonometric Function/1
  Demux/2 -> Mux/2
  Demux/3 -> Mux/3
  Gain5/1 -> r_1/1
  Normalize Vector1/1 -> rw_lat x ez1/1(a(1) a(2) a(3)), e_long1/1
  ez 1/1 -> Mux/1

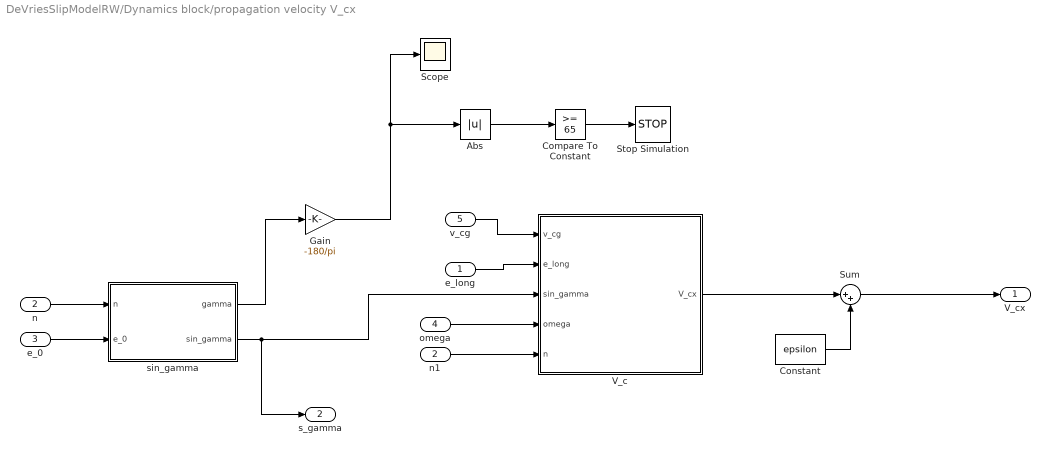
== system DeVriesSlipModelRW/Dynamics block/propagation velocity V_cx ==
  e_long : Inport
  n : Inport  Port=2
  e_0 : Inport  Port=3
  omega : Inport  Port=4
  v_cg : Inport  Port=5
  Abs : Abs
  Compare To Constant : simulink/Logic and Bit Operations/Compare To Constant  relop=>=  const=65  OutDataTypeStr=boolean
  Constant : Constant  Value=epsilon
  Gain : Gain  Gain=-180/pi
  Scope : Scope
  Stop Simulation : Stop
  Sum : Sum  Inputs=|++
  V_c : Subsystem
  n1 : InportShadow  Port=2
  sin_gamma : Subsystem
  V_cx : Outport
  s_gamma : Outport  Port=2
  wires:
  n/1 -> sin_gamma/1(n)
  e_0/1 -> sin_gamma/2(e_0)
  sin_gamma/1(gamma) -> Gain/1
  v_cg/1 -> V_c/1(v_cg)
  e_long/1 -> V_c/2(e_long)
  sin_gamma/2(sin_gamma) -> s_gamma/1, V_c/3(sin_gamma)
  omega/1 -> V_c/4(omega)
  n1/1 -> V_c/5(n)
  Gain/1 -> Scope/1, Abs/1
  Compare To Constant/1 -> Stop Simulation/1
  Abs/1 -> Compare To Constant/1
  V_c/1(V_cx) -> Sum/1
  Sum/1 -> V_cx/1
  Constant/1 -> Sum/2

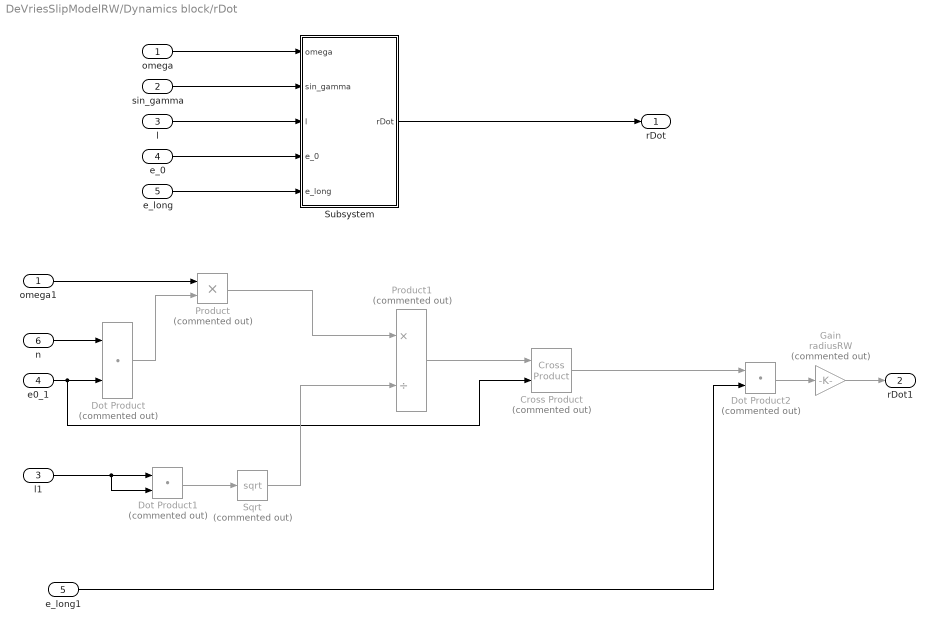
== system DeVriesSlipModelRW/Dynamics block/rDot ==
  omega : Inport
  sin_gamma : Inport  Port=2
  l : Inport  Port=3
  e_0 : Inport  Port=4
  e_long : Inport  Port=5
  n : Inport  Port=6
  Cross Product : Contact_Forces_Lib/Math/Cross Product  Commented=on
  Dot Product : DotProduct  Commented=on  InputSameDT=on  OutDataTypeStr=Inherit: Inherit via internal rule
  Dot Product1 : DotProduct  Commented=on  InputSameDT=on  OutDataTypeStr=Inherit: Inherit via internal rule
  Dot Product2 : DotProduct  Commented=on  InputSameDT=on  OutDataTypeStr=Inherit: Inherit via internal rule
  Gain : Gain  Commented=on  Gain=radiusRW
  Product : Product  Commented=on
  Product1 : Product  Commented=on  Inputs=*/
  Sqrt : Sqrt  Commented=on  SaturateOnIntegerOverflow=on
  Subsystem : Subsystem
  e0_1 : InportShadow  Port=4
  e_long1 : InportShadow  Port=5
  l1 : InportShadow  Port=3
  omega1 : InportShadow
  rDot : Outport
  rDot1 : Outport  Port=2
  wires:
  omega/1 -> Subsystem/1(omega)
  sin_gamma/1 -> Subsystem/2(sin_gamma)
  l/1 -> Subsystem/3(l)
  e_0/1 -> Subsystem/4(e_0)
  e_long/1 -> Subsystem/5(e_long)
  Subsystem/1(rDot) -> rDot/1
  omega1/1 -> Product/1
  n/1 -> Dot Product/1
  e0_1/1 -> Cross Product/2, Dot Product/2
  Dot Product/1 -> Product/2
  Product/1 -> Product1/1
  Dot Product1/1 -> Sqrt/1
  l1/1 -> Dot Product1/2, Dot Product1/1
  Sqrt/1 -> Product1/2
  e_long1/1 -> Dot Product2/2
  Dot Product2/1 -> Gain/1
  Gain/1 -> rDot1/1
  Product1/1 -> Cross Product/1
  Cross Product/1 -> Dot Product2/1

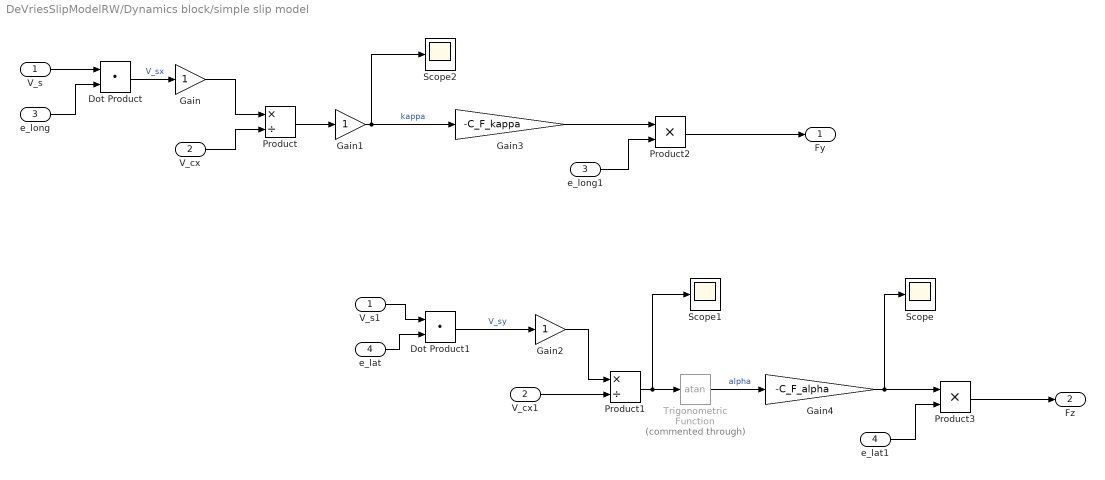
== system DeVriesSlipModelRW/Dynamics block/simple slip model ==
  V_s : Inport
  V_cx : Inport  Port=2
  e_long : Inport  Port=3
  e_lat : Inport  Port=4
  Dot Product : DotProduct  InputSameDT=on  OutDataTypeStr=Inherit: Inherit via internal rule
  Dot Product1 : DotProduct  InputSameDT=on  OutDataTypeStr=Inherit: Inherit via internal rule
  Gain : Gain
  Gain1 : Gain
  Gain2 : Gain
  Gain3 : Gain  Gain=-C_F_kappa
  Gain4 : Gain  Gain=-C_F_alpha
  Product : Product  Inputs=*/
  Product1 : Product  Inputs=*/
  Product2 : Product
  Product3 : Product
  Scope : Scope
  Scope1 : Scope
  Scope2 : Scope
  Trigonometric Function : Trigonometry  Commented=through  Operator=atan
  V_cx1 : InportShadow  Port=2
  V_s1 : InportShadow
  e_lat1 : InportShadow  Port=4
  e_long1 : InportShadow  Port=3
  Fy : Outport
  Fz : Outport  Port=2
  wires:
  V_s/1 -> Dot Product/1
  e_long/1 -> Dot Product/2
  Dot Product/1 -> Gain/1  "V_sx"
  Gain/1 -> Product/1
  Product/1 -> Gain1/1
  Gain1/1 -> Scope2/1, Gain3/1  "kappa"
  V_s1/1 -> Dot Product1/1
  e_lat/1 -> Dot Product1/2
  Dot Product1/1 -> Gain2/1  "V_sy"
  Gain2/1 -> Product1/1
  Product1/1 -> Scope1/1, Trigonometric Function/1
  Trigonometric Function/1 -> Gain4/1  "alpha"
  e_long1/1 -> Product2/2
  e_lat1/1 -> Product3/2
  Gain3/1 -> Product2/1
  Product2/1 -> Fy/1
  Gain4/1 -> Scope/1, Product3/1
  Product3/1 -> Fz/1
  V_cx1/1 -> Product1/2
  V_cx/1 -> Product/2

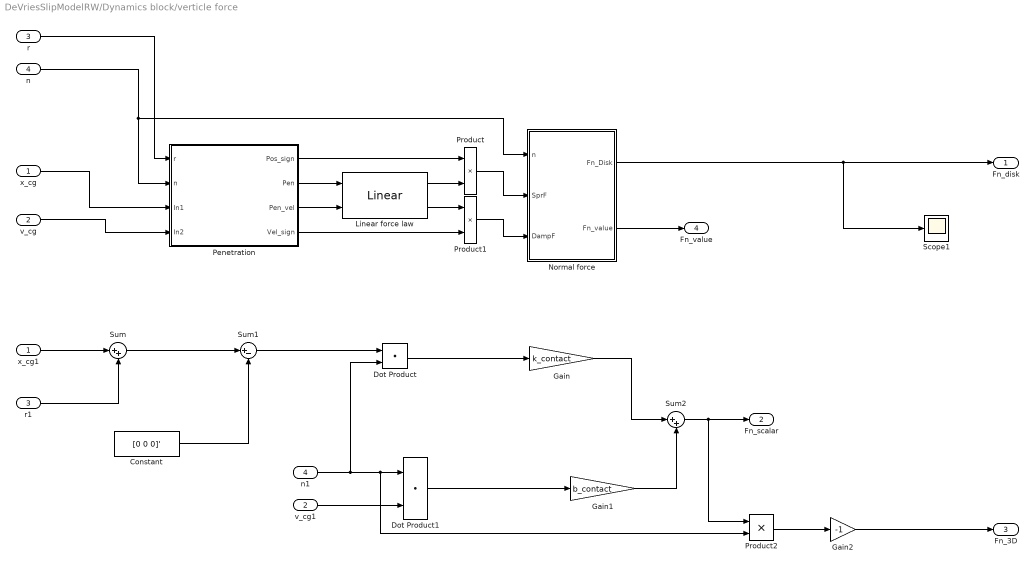
== system DeVriesSlipModelRW/Dynamics block/verticle force ==
  x_cg : Inport
  v_cg : Inport  Port=2
  r : Inport  Port=3
  n : Inport  Port=4
  Constant : Constant  Value=[0 0 0]'
  Dot Product : DotProduct  InputSameDT=on  OutDataTypeStr=Inherit: Inherit via internal rule
  Dot Product1 : DotProduct  InputSameDT=on  OutDataTypeStr=Inherit: Inherit via internal rule
  Gain : Gain  Gain=k_contact
  Gain1 : Gain  Gain=b_contact
  Gain2 : Gain  Gain=-1
  Linear force law : Contact_Forces_Lib/Force Law/Linear  VariantControl=Linear  k_pen=k_contact  b_penvel=b_contact
  Normal force : Subsystem
  Penetration : Subsystem
  Product : Product
  Product1 : Product
  Product2 : Product
  Scope1 : Scope
  Sum : Sum  Inputs=|++
  Sum1 : Sum  Inputs=|+-
  Sum2 : Sum  Inputs=|++
  n1 : InportShadow  Port=4
  r1 : InportShadow  Port=3
  v_cg1 : InportShadow  Port=2
  x_cg1 : InportShadow
  Fn_disk : Outport
  Fn_scalar : Outport  Port=2
  Fn_3D : Outport  Port=3
  Fn_value : Outport  Port=4
  wires:
  x_cg/1 -> Penetration/3(In1)
  v_cg/1 -> Penetration/4(In2)
  Penetration/2(Pen) -> Linear force law/1
  Penetration/3(Pen_vel) -> Linear force law/2
  Linear force law/1 -> Product/2
  Penetration/1(Pos_sign) -> Product/1
  Linear force law/2 -> Product1/1
  Penetration/4(Vel_sign) -> Product1/2
  Product/1 -> Normal force/2(SprF)
  Product1/1 -> Normal force/3(DampF)
  Normal force/1(Fn_Disk) -> Scope1/1, Fn_disk/1
  n/1 -> Normal force/1(n), Penetration/2(n)
  r/1 -> Penetration/1(r)
  x_cg1/1 -> Sum/1
  r1/1 -> Sum/2
  Sum/1 -> Sum1/1
  Constant/1 -> Sum1/2
  Sum1/1 -> Dot Product/1
  n1/1 -> Product2/2, Dot Product1/1, Dot Product/2
  Dot Product/1 -> Gain/1
  v_cg1/1 -> Dot Product1/2
  Dot Product1/1 -> Gain1/1
  Gain/1 -> Sum2/1
  Gain1/1 -> Sum2/2
  Sum2/1 -> Product2/1, Fn_scalar/1
  Product2/1 -> Gain2/1
  Gain2/1 -> Fn_3D/1
  Normal force/2(Fn_value) -> Fn_value/1

== system DeVriesSlipModelRW/Dynamics block/Wheel_vector_calculation/rw_lat x ez ==
  a(1) a(2) a(3) : Inport
  b(1) b(2) b(3) : Inport  Port=2
  Product : Product  SaturateOnIntegerOverflow=on  RndMeth=Zero  InputSameDT=on  OutDataTypeStr=Inherit: Same as first input
  Product1 : Product  SaturateOnIntegerOverflow=on  RndMeth=Zero  InputSameDT=on  OutDataTypeStr=Inherit: Same as first input
  Selector : Selector  InputPortWidth=3  IndexOptions=Index vector (dialog)  Indices=[2 3 1]  OutputSizes=1
  Selector1 : Selector  InputPortWidth=3  IndexOptions=Index vector (dialog)  Indices=[3 1 2]  OutputSizes=1
  Selector2 : Selector  InputPortWidth=3  IndexOptions=Index vector (dialog)  Indices=[2 3 1]  OutputSizes=1
  Selector3 : Selector  InputPortWidth=3  IndexOptions=Index vector (dialog)  Indices=[3 1 2]  OutputSizes=1
  Sum : Sum  Inputs=+|-  SaturateOnIntegerOverflow=on  InputSameDT=on  OutDataTypeStr=Inherit: Same as first input
  c(1) c(2) c(3) : Outport  InitialOutput=0
  wires:
  Sum/1 -> c(1) c(2) c(3)/1
  b(1) b(2) b(3)/1 -> Selector1/1, Selector2/1
  Selector/1 -> Product/1
  a(1) a(2) a(3)/1 -> Selector/1, Selector3/1
  Product/1 -> Sum/1
  Selector1/1 -> Product/2
  Product1/1 -> Sum/2
  Selector2/1 -> Product1/2
  Selector3/1 -> Product1/1

== system DeVriesSlipModelRW/Dynamics block/Wheel_vector_calculation/rw_lat x ez1 ==
  a(1) a(2) a(3) : Inport
  b(1) b(2) b(3) : Inport  Port=2
  Product : Product  SaturateOnIntegerOverflow=on  RndMeth=Zero  InputSameDT=on  OutDataTypeStr=Inherit: Same as first input
  Product1 : Product  SaturateOnIntegerOverflow=on  RndMeth=Zero  InputSameDT=on  OutDataTypeStr=Inherit: Same as first input
  Selector : Selector  InputPortWidth=3  IndexOptions=Index vector (dialog)  Indices=[2 3 1]  OutputSizes=1
  Selector1 : Selector  InputPortWidth=3  IndexOptions=Index vector (dialog)  Indices=[3 1 2]  OutputSizes=1
  Selector2 : Selector  InputPortWidth=3  IndexOptions=Index vector (dialog)  Indices=[2 3 1]  OutputSizes=1
  Selector3 : Selector  InputPortWidth=3  IndexOptions=Index vector (dialog)  Indices=[3 1 2]  OutputSizes=1
  Sum : Sum  Inputs=+|-  SaturateOnIntegerOverflow=on  InputSameDT=on  OutDataTypeStr=Inherit: Same as first input
  c(1) c(2) c(3) : Outport  InitialOutput=0
  wires:
  Selector3/1 -> Product1/1
  Selector2/1 -> Product1/2
  Product1/1 -> Sum/2
  Selector1/1 -> Product/2
  Product/1 -> Sum/1
  a(1) a(2) a(3)/1 -> Selector3/1, Selector/1
  Selector/1 -> Product/1
  b(1) b(2) b(3)/1 -> Selector2/1, Selector1/1
  Sum/1 -> c(1) c(2) c(3)/1

== system DeVriesSlipModelRW/Dynamics block/propagation velocity V_cx/V_c ==
  v_cg : Inport
  e_long : Inport  Port=2
  sin_gamma : Inport  Port=3
  omega : Inport  Port=4
  n : Inport  Port=5
  Dot Product : DotProduct  InputSameDT=on  OutDataTypeStr=Inherit: Inherit via internal rule
  Dot Product2 : DotProduct  InputSameDT=on  OutDataTypeStr=Inherit: Inherit via internal rule
  Gain : Gain  Gain=radiusRW
  Product : Product
  Sum : Sum  Inputs=|++
  V_cx : Outport
  wires:
  n/1 -> Dot Product/2
  Gain/1 -> Product/1
  Product/1 -> Sum/2
  Dot Product2/1 -> V_cx/1  "V_cx"
  Sum/1 -> Dot Product2/1  "V_c"
  Dot Product/1 -> Product/2  "psiDot"
  sin_gamma/1 -> Gain/1
  omega/1 -> Dot Product/1
  e_long/1 -> Dot Product2/2
  v_cg/1 -> Sum/1

== system DeVriesSlipModelRW/Dynamics block/propagation velocity V_cx/sin_gamma ==
  n : Inport
  e_0 : Inport  Port=2
  Dot Product : DotProduct  InputSameDT=on  OutDataTypeStr=Inherit: Inherit via internal rule
  Trigonometric Function : Trigonometry  Operator=asin
  gamma : Outport
  sin_gamma : Outport  Port=2
  wires:
  n/1 -> Dot Product/1
  Trigonometric Function/1 -> gamma/1
  e_0/1 -> Dot Product/2
  Dot Product/1 -> sin_gamma/1, Trigonometric Function/1  "sin_gamma"

== system DeVriesSlipModelRW/Dynamics block/rDot/Subsystem ==
  omega : Inport
  sin_gamma : Inport  Port=2
  l : Inport  Port=3
  e_0 : Inport  Port=4
  e_long : Inport  Port=5
  Cross Product : Contact_Forces_Lib/Math/Cross Product
  Dot Product : DotProduct  InputSameDT=on  OutDataTypeStr=Inherit: Inherit via internal rule
  Dot Product1 : DotProduct  InputSameDT=on  OutDataTypeStr=Inherit: Inherit via internal rule
  Product : Product
  Product1 : Product  Inputs=*/
  Sqrt : Sqrt  SaturateOnIntegerOverflow=on
  rDot : Outport
  wires:
  sin_gamma/1 -> Product/2
  Cross Product/1 -> Dot Product1/1
  e_long/1 -> Dot Product1/2
  omega/1 -> Product/1
  Dot Product1/1 -> rDot/1
  Product/1 -> Product1/1
  Dot Product/1 -> Sqrt/1
  l/1 -> Dot Product/2, Dot Product/1
  Sqrt/1 -> Product1/2
  Product1/1 -> Cross Product/1
  e_0/1 -> Cross Product/2

== system DeVriesSlipModelRW/Dynamics block/verticle force/Normal force ==
  n : Inport
  SprF : Inport  Port=2
  DampF : Inport  Port=3
  Add : Sum
  Product : Product
  Fn_Disk : Outport
  Fn_value : Outport  Port=2
  wires:
  SprF/1 -> Add/1
  DampF/1 -> Add/2
  Add/1 -> Fn_value/1, Product/1
  n/1 -> Product/2
  Product/1 -> Fn_Disk/1

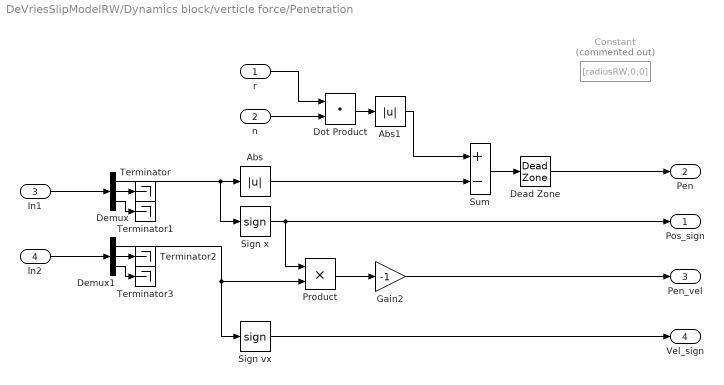
== system DeVriesSlipModelRW/Dynamics block/verticle force/Penetration ==
  r : Inport
  n : Inport  Port=2
  In1 : Inport  Port=3
  In2 : Inport  Port=4
  Abs : Abs  ZeroCross=off
  Abs1 : Abs
  Constant : Constant  Commented=on  Value=[radiusRW;0;0]
  Dead Zone : DeadZone  LowerValue=-inf  UpperValue=0  SaturateOnIntegerOverflow=on
  Demux : Demux  Outputs=3
  Demux1 : Demux  Outputs=3
  Dot Product : DotProduct  InputSameDT=on  OutDataTypeStr=Inherit: Inherit via internal rule
  Gain2 : Gain  Gain=-1
  Product : Product
  Sign vx : Signum  ZeroCross=off
  Sign x : Signum  ZeroCross=off
  Sum : Sum  Inputs=+-
  Terminator{,1..3} (4 alike) : Terminator
  Pos_sign : Outport
  Pen : Outport  Port=2
  Pen_vel : Outport  Port=3
  Vel_sign : Outport  Port=4
  wires:
  Demux1/3 -> Terminator3/1
  Demux/2 -> Terminator/1
  Gain2/1 -> Pen_vel/1
  Dead Zone/1 -> Pen/1
  Sign x/1 -> Pos_sign/1, Product/1
  Demux1/1 -> Product/2, Sign vx/1
  Abs/1 -> Sum/2
  Product/1 -> Gain2/1
  Sign vx/1 -> Vel_sign/1
  Demux/1 -> Sign x/1, Abs/1
  Sum/1 -> Dead Zone/1
  Demux/3 -> Terminator1/1
  Demux1/2 -> Terminator2/1
  In1/1 -> Demux/1
  In2/1 -> Demux1/1
  n/1 -> Dot Product/2
  Dot Product/1 -> Abs1/1
  r/1 -> Dot Product/1
  Abs1/1 -> Sum/1
